simulink model "Pierwsza_metoda"  (R2022a)
settings: Solver=VariableStepAuto  StartTime=0.0  StopTime=50  RelTol=1e-3
settings Model: Creator=danie  LastModifiedBy=danie

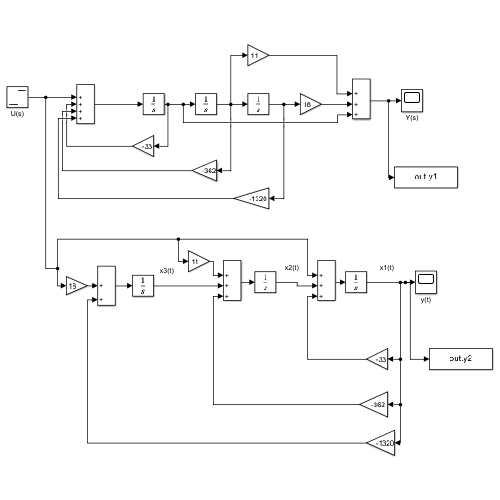
[thumbnail: Simulink's stored preview of the top-level diagram]
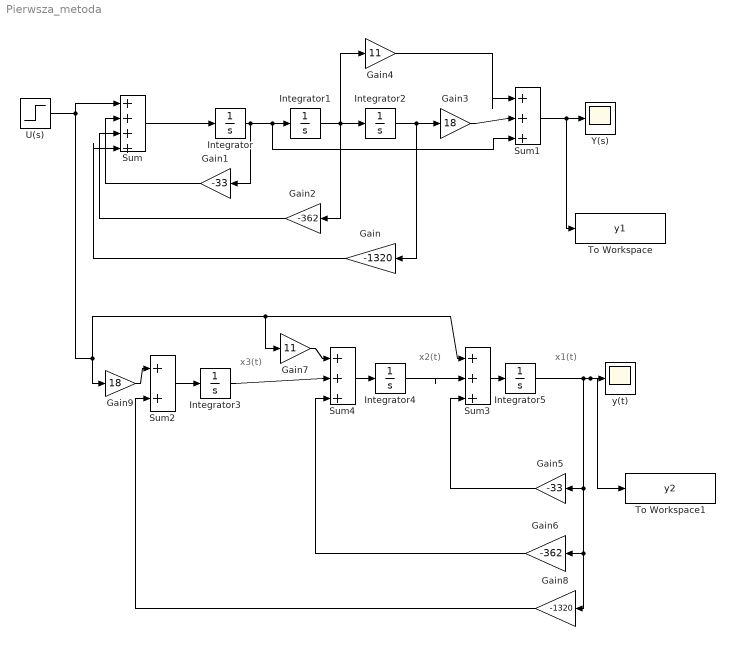
== system Pierwsza_metoda ==
  note: x1(t)
  note: x3(t)
  note: x2(t)
  Gain : Gain  Gain=-1320
  Gain1 : Gain  Gain=-33
  Gain2 : Gain  Gain=-362
  Gain3 : Gain  Gain=18
  Gain4 : Gain  Gain=11
  Gain5 : Gain  Gain=-33
  Gain6 : Gain  Gain=-362
  Gain7 : Gain  Gain=11
  Gain8 : Gain  Gain=-1320
  Gain9 : Gain  Gain=18
  Integrator : Integrator  InitialCondition=1
  Integrator1 : Integrator  InitialCondition=-1
  Integrator2 : Integrator  InitialCondition=2
  Integrator3 : Integrator
  Integrator4 : Integrator
  Integrator5 : Integrator
  Sum : Sum  Inputs=|++++
  Sum1 : Sum  Inputs=|+++
  Sum2 : Sum  Inputs=|++
  Sum3 : Sum  Inputs=|+++
  Sum4 : Sum  Inputs=|+++
  To Workspace : ToWorkspace  VariableName=y1  SaveFormat=Structure With Time  SampleTime=-1
  To Workspace1 : ToWorkspace  VariableName=y2  SaveFormat=Structure With Time  SampleTime=-1
  U(s) : Step  SampleTime=0
  Y(s) : Scope
  y(t) : Scope
  wires:
  Sum/1 -> Integrator/1
  Integrator/1 -> Gain1/1, Sum1/3, Integrator1/1
  Integrator1/1 -> Gain4/1, Gain2/1, Integrator2/1
  Sum1/1 -> To Workspace/1, Y(s)/1
  Gain1/1 -> Sum/2
  Gain2/1 -> Sum/3
  Integrator2/1 -> Gain/1, Gain3/1
  Gain3/1 -> Sum1/2
  Gain/1 -> Sum/4
  Gain4/1 -> Sum1/1
  Gain8/1 -> Sum2/2
  Integrator3/1 -> Sum4/2
  Sum4/1 -> Integrator4/1
  Gain6/1 -> Sum4/3
  Gain7/1 -> Sum4/1
  Integrator4/1 -> Sum3/2
  Gain9/1 -> Sum2/1
  Integrator5/1 -> Gain8/1, Gain6/1, Gain5/1, To Workspace1/1, y(t)/1
  Sum3/1 -> Integrator5/1
  Gain5/1 -> Sum3/3
  U(s)/1 -> Gain9/1, Sum3/1, Gain7/1, Sum/1
  Sum2/1 -> Integrator3/1
